simulink model "InteresAhorro"  (R2023b)
settings: Solver=FixedStepDiscrete  StartTime=0.0  StopTime=5  RelTol=1e-3
settings Model: Creator=alfre  LastModifiedBy=alfre

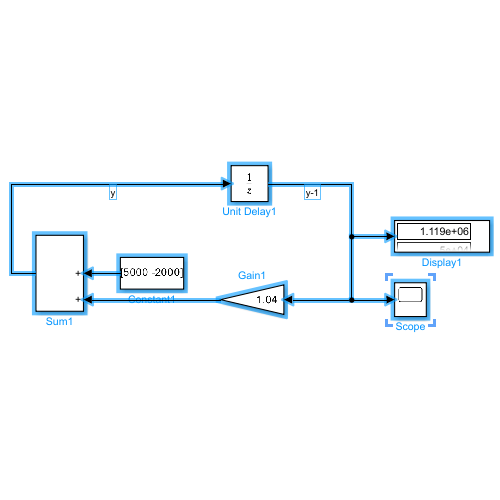
[thumbnail: Simulink's stored preview of the top-level diagram]
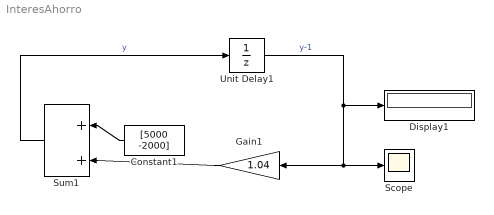
== system InteresAhorro ==
  Constant1 : Constant  Value=[5000 -2000]
  Display1 : Display
  Gain1 : Gain  Gain=1.04
  Scope : Scope
  Sum1 : Sum  Inputs=|++
  Unit Delay1 : UnitDelay  InitialCondition=50000  SampleTime=-1  HasFrameUpgradeWarning=on
  wires:
  Gain1/1 -> Sum1/2
  Unit Delay1/1 -> Display1/1, Scope/1, Gain1/1  "y-1"
  Sum1/1 -> Unit Delay1/1  "y"
  Constant1/1 -> Sum1/1
